simulink model "DecoupledSimulator"  (R2023b)
settings: Solver=FixedStepAuto  StartTime=0.0  StopTime=100.0  FixedStep=0.05  MaxStep=0.1  MinStep=5e-2  RelTol=1e-3
values from neighbouring files (symbols this model uses):
  p = c2d(ss(A,B,C,D),0.05)    [YalmipMpc.m]
undefined symbols (not defined in the file or in its folder): initialconditions, k, Sat_dyn_Lin_Decoupled, YalmipMpc
libraries: mpclib x1
settings Model: SimulationMode=accelerator  Creator=simone  LastModifiedBy=simone
settings ModelReferenceCC: UpdateModelReferenceTargets=Force

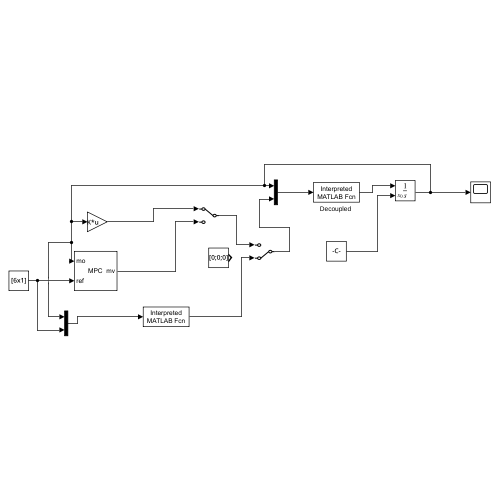
[thumbnail: Simulink's stored preview of the top-level diagram]
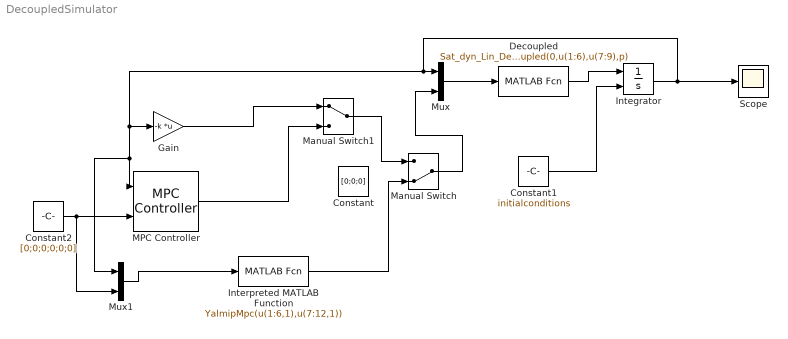
== system DecoupledSimulator ==
  Constant : Constant  Value=[0;0;0]
  Constant1 : Constant  Value=initialconditions  VectorParams1D=off
  Constant2 : Constant  Value=[0;0;0;0;0;0]
  "Decoupled " : MATLABFcn  MATLABFcn=Sat_dyn_Lin_Decoupled(0,u(1:6),u(7:9),p)  OutputDimensions=6  OutputSignalType=real
  Gain : Gain  Gain=-k  Multiplication=Matrix(K*u)
  Integrator : Integrator  InitialConditionSource=external  InitialCondition=initialconditions
  Interpreted MATLAB Function : MATLABFcn  MATLABFcn=YalmipMpc(u(1:6,1),u(7:12,1))  OutputDimensions=3
  MPC Controller : mpclib/MPC Controller  SCDEnableBlockLinearizationSpecification=on  is_multiple=0  enable_value=0  return_u0=off  updateMPCinCallerWorkspace=on  md_inport=off  mv_inport=off  uref_inport=off  return_cost=off  return_mvseq=off  return_qpstatus=off  return_xseq=off  return_state=off  return_ovseq=off  state_inport=off  umin_inport=off  umax_inport=off  ymin_inport=off  ymax_inport=off  cc_inport=off  ywt_inport=off  uwt_inport=off  duwt_inport=off  rhoeps_inport=off  pm_inport=off  MaximumP=10  HorizonChoice=FixedHorizon  n_ts=1  n_p=7  n_mv=3  n_md=0  n_ud=0  n_mo=6  n_uo=0  BlockDataType=double  SampleTimeInherited=off  switch_inport=off
  Manual Switch : ManualSwitch  CurrentSetting=0
  Manual Switch1 : ManualSwitch
  Mux : Mux  Inputs=2
  Mux1 : Mux  Inputs=2
  Scope : Scope
  wires:
  Integrator/1 -> Scope/1, Mux1/1, MPC Controller/1, Gain/1, Mux/1
  "Decoupled "/1 -> Integrator/1
  Mux/1 -> "Decoupled "/1
  Gain/1 -> Manual Switch1/1
  Manual Switch/1 -> Mux/2
  Constant1/1 -> Integrator/2
  Manual Switch1/1 -> Manual Switch/1
  MPC Controller/1 -> Manual Switch1/2
  Constant2/1 -> Mux1/2, MPC Controller/2
  Mux1/1 -> Interpreted MATLAB Function/1
  Interpreted MATLAB Function/1 -> Manual Switch/2
